simulink model "Pedestrian_Detection_CS2018"  (R2017a)
settings: Solver=ode45  StartTime=0  StopTime=11  FixedStep=0.001  RelTol=1e-3  AbsTol=1e-6
undefined symbols (not defined in the file): gray
libraries: Solver_SF x2
settings Model: ExtModeTrigMode=oneshot  ExtModeArmWhenConnect=off  Creator=ywata  LastModifiedBy=jhu
settings DataIOCC: SaveFormat=Array  SignalLoggingSaveFormat=ModelDataLogs  SignalLoggingName=sigsOut
settings OptimizationCC: BlockReduction=off  BooleanDataType=off  LifeSpan=inf
settings DebuggingCC: SaveWithParameterizedLinksMsg=none  UnderspecifiedInitializationDetection=Classic  MergeDetectMultiDrivingBlocksExec=none  SignalResolutionControl=TryResolveAllWithWarning  InheritedTsInSrcMsg=none  MultiTaskDSMMsg=warning  MultiTaskCondExecSysMsg=none  FcnCallInpInsideContextMsg=warning  StateNameClashWarn=warning  SFUnexpectedBacktrackingDiag=warning  SFNoUnconditionalDefaultTransitionDiag=warning  SFExecutionAtInitializationDiag=none
settings HardwareCC: ProdBitPerPointer=32  ProdBitPerSizeT=32  ProdBitPerPtrDiffT=32  ProdLargestAtomicFloat=None  ProdIntDivRoundTo=Undefined  ProdEndianess=Unspecified  ProdWordSize=32  ProdHWDeviceType=32-bit Generic  TargetBitPerPointer=64  TargetBitPerSizeT=64  TargetBitPerPtrDiffT=64  TargetLongLongMode=on  TargetIntDivRoundTo=Zero  TargetEndianess=LittleEndian  TargetWordSize=64  TargetHWDeviceType=MATLAB Host  ProdEqTarget=off
settings ModelReferenceCC: PropagateSignalLabelsOutOfModel=off
settings RTWCC: TemplateMakefile=grt_vc.tmf
settings GRTTargetCC: TargetFcnLib=ansi_tfl_tmw.mat  TargetLangStandard=C89/C90 (ANSI)  CombineOutputUpdateFcns=off  GRTInterface=on
settings ConfigComp: CovMetricSettings=dw  CovHtmlReporting=on  CovSaveCumulativeToWorkspaceVar=on  CovSaveSingleToWorkspaceVar=on  CovExternalEMLEnable=off

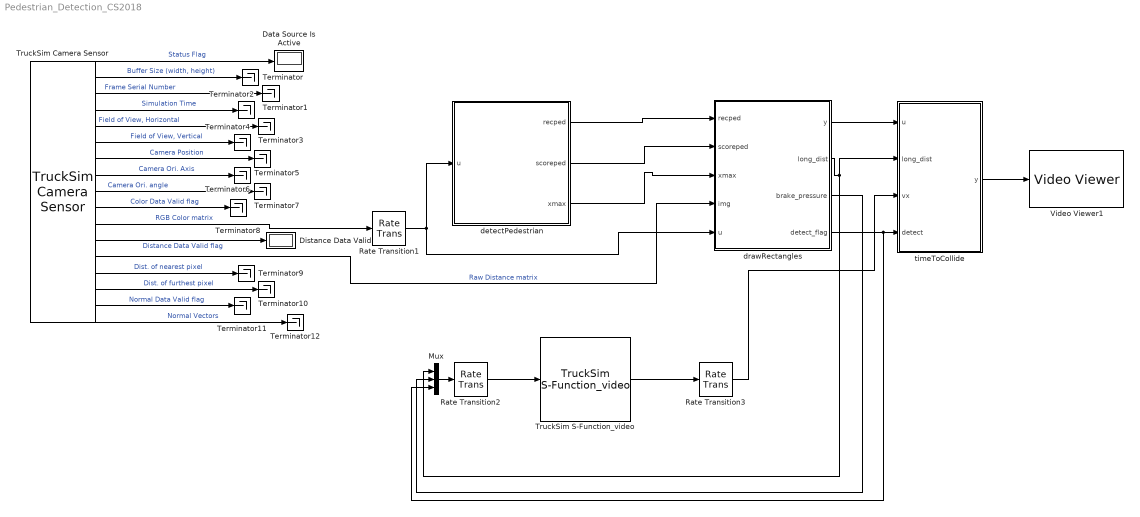
== system Pedestrian_Detection_CS2018 ==
  Data Source Is Active : Display
  Distance Data Valid : Display
  Mux : Mux  Inputs=3
  Rate Transition1 : RateTransition  OutPortSampleTime=0.05
  Rate Transition2 : RateTransition  OutPortSampleTime=0.05
  Rate Transition3 : RateTransition  OutPortSampleTime=0.05
  Terminator{,1..12} (13 alike) : Terminator
  TruckSim Camera Sensor : Solver_SF/TruckSim Camera Sensor
  TruckSim S-Function_video : Solver_SF/TruckSim S-Function_video  Priority=1  SIMFILE=simfile.sim
  "Video Viewer1 " : VideoViewer  colormapValue=gray(256)  FigPos=[1373 439 425 224]
  detectPedestrian : MATLAB Function  TreatAsAtomicUnit=on
  drawRectangles : MATLAB Function  TreatAsAtomicUnit=on
  timeToCollide : MATLAB Function  TreatAsAtomicUnit=on
  wires:
  TruckSim Camera Sensor/11 -> Rate Transition1/1  "RGB Color matrix"
  TruckSim Camera Sensor/1 -> Data Source Is Active/1  "Status Flag"
  TruckSim Camera Sensor/17 -> Terminator12/1  "Normal Vectors"
  TruckSim Camera Sensor/2 -> Terminator/1  "Buffer Size (width, height)"
  TruckSim Camera Sensor/14 -> Terminator9/1  "Dist. of nearest pixel"
  TruckSim Camera Sensor/15 -> Terminator10/1  "Dist. of furthest pixel"
  TruckSim Camera Sensor/16 -> Terminator11/1  "Normal Data Valid flag"
  TruckSim Camera Sensor/12 -> Distance Data Valid/1  "Distance Data Valid flag"
  TruckSim Camera Sensor/10 -> Terminator8/1  "Color Data Valid flag"
  TruckSim Camera Sensor/3 -> Terminator1/1  "Frame Serial Number"
  TruckSim Camera Sensor/4 -> Terminator2/1  "Simulation Time"
  TruckSim Camera Sensor/5 -> Terminator3/1  "Field of View, Horizontal"
  TruckSim Camera Sensor/6 -> Terminator4/1  "Field of View, Vertical"
  TruckSim Camera Sensor/7 -> Terminator5/1  "Camera Position"
  TruckSim Camera Sensor/8 -> Terminator6/1  "Camera Ori. Axis"
  TruckSim Camera Sensor/9 -> Terminator7/1  "Camera Ori. angle"
  detectPedestrian/1(recped) -> drawRectangles/1(recped)
  detectPedestrian/2(scoreped) -> drawRectangles/2(scoreped)
  TruckSim Camera Sensor/13 -> drawRectangles/4(img)  "Raw Distance matrix"
  Rate Transition1/1 -> drawRectangles/5(u), detectPedestrian/1(u)
  drawRectangles/1(y) -> timeToCollide/1(u)
  detectPedestrian/3(xmax) -> drawRectangles/3(xmax)
  Mux/1 -> Rate Transition2/1
  drawRectangles/3(brake_pressure) -> Mux/2
  drawRectangles/2(long_dist) -> Mux/1, timeToCollide/2(long_dist)
  Rate Transition2/1 -> TruckSim S-Function_video/1
  TruckSim S-Function_video/1 -> Rate Transition3/1
  timeToCollide/1(y) -> "Video Viewer1 "/1
  Rate Transition3/1 -> timeToCollide/3(vx)
  drawRectangles/4(detect_flag) -> Mux/3, timeToCollide/4(detect)

== matlab function Pedestrian_Detection_CS2018/drawRectangles ==
  data: recped input; scoreped input; xmax input; img input; u input; y output; long_dist output; brake_pressure output; detect_flag output
function [y, long_dist, brake_pressure, detect_flag] = drawRectangles(recped, scoreped, xmax, img, u)

% img = distance matrix image
% u = RGB matrix image

coder.extrinsic('sprintf')
tmax = length(scoreped);

y = u;

long_dist = 10000;
detect_flag = 0;

% the following value need to be changed according to
% the vehicle. This value is defined in TruckSim. 
axle_track = 1.750;
% randomly selected the lateral safe distance.
safety_dist = axle_track*2;
% assuming the field of view is 55.  This is defined
% in CarSim.  change the following value if necessary.
fov = 55.0;
half_fov = fov/2;
[tot_row, tot_col] = size(img);

brake_pressure = 0;
j = 1;
if xmax > 0    
    if (xmax == 1)
      j = 1;
    end
    % if we want to deal with multiple pedestrian, need to change
    % the following lines.  maybe need to add a loop to process
    % each pedestrian. probably need to check the x y location to see
    % if the objects are too close to each other.
    if (xmax > 1)
      [M,I] = max(scoreped(:));
      j = 1;
    end
    width = recped(j,3);
    height = recped(j,4);
    rect = [recped(j,1) recped(j,2) width height];
    y=insertShape(y, 'rectangle', rect, 'LineWidth', 1);
    text_pos = [recped(j,1), recped(j,2)-20];
    conf = sprintf('Confidence: %0.1f %', scoreped(j));

    row = rect(2) + ceil(height/2);
    col = rect(1) + ceil(width/2);
    pix = [row col];
    pix_dist = double(img(pix(1),pix(2)));
    lat_pix = abs(col/2 - pix(2));
    ang_pix = single(lat_pix*half_fov/(tot_col/2));
    lat_dist = pix_dist*tan(ang_pix/180*pi);
    %long_dist = double(pix_dist*cos(ang_pix/180*pi));
    long_dist = double(pix_dist);
    
    text_pos = [10, 10];
    dist_text = sprintf('Distance: %0.2f m', long_dist);
    y=insertText(y, text_pos, dist_text, 'FontSize', 12);
    
    if (long_dist < 8.0) && (lat_dist < safety_dist) 
        brake_pressure = 100;
    end
    
    detect_flag = 1;
    
end

== matlab function Pedestrian_Detection_CS2018/detectPedestrian ==
  data: recped output; scoreped output; xmax output; u input
function [recped, scoreped, xmax] = detectPedestrian(u)

recped = zeros(10,4);
scoreped = zeros(10,1);

coder.extrinsic('peopleDetectorACF');
coder.extrinsic('detect');
detector=peopleDetectorACF('caltech');


roi = [1 1 300 180]; % use the whole screen for now.
%roi = [1 120 300 370]
resizeRatio = 1.5;
frame = imresize(u, resizeRatio, 'Antialiasing', false);

[bboxes, scores] = detect(detector, u, roi, ...
    'WindowStride', 2, ...
    'NumScaleLevels', 32, ...
    'SelectStrongest', false);

xmax = 0;
col = 0;
row = 0;
xmax = length(scores);

if xmax > 10
    xmax = 10;
end
if xmax > 0
    for i=1:xmax
        recped(i,1) = bboxes(i,1);
        recped(i,2) = bboxes(i,2);
        recped(i,3) = bboxes(i,3);
        recped(i,4) = bboxes(i,4);
        scoreped(i) = scores(i);
    end
end
%
%y = u;

== matlab function Pedestrian_Detection_CS2018/timeToCollide ==
  data: u input; y output; long_dist input; vx input; detect input
function y = Time_To_Collision(u, long_dist, vx, detect)

coder.extrinsic('sprintf')
y = u;
% convert km/h to m/s
vel = vx*1000/3600;
time_to_collide = long_dist/vx;

% may or may not need to put vel > 1.0 m/s. adjust this for your project.
if (detect > 0) && (time_to_collide > 0) && (vel > 1)
    text_pos2 = [10, 30];
    time_text = sprintf('Time to Collision: %0.2f s' ,time_to_collide);
    y = insertText(y, text_pos2, time_text, 'FontSize', 12);
end
